simulink model "TEST_IPM_2_0"  (R2019b)
settings: configuration reference "Configuration" (kept outside this file)
PreLoadFcn:
  | RTWConfigurationCB('preloadfcn', bdroot);
values from neighbouring files (symbols this model uses):
  MParamFbase = 200.0    [TEST_IPM_LIB.sldd]
  MParamIbase = 360.0    [TEST_IPM_LIB.sldd]
  MParamLd = 0.002    [TEST_IPM_LIB.sldd]
  MParamLq = 0.002    [TEST_IPM_LIB.sldd]
  MParamRs = 1.15    [TEST_IPM_LIB.sldd]
  PWM_TPBRD_HALF = 5000.0    [TEST_IPM_LIB.sldd]
  Ts_10kHz = 0.0001    [TEST_IPM_LIB.sldd]
  Ts_1kHz = 0.001    [TEST_IPM_LIB.sldd]
undefined symbols (not defined in the file or in its folder): Down, GPTRIP1SEL, GPTRIP2SEL, TZ1, TZ2, Up
libraries: c280xlib x66, c2837xDlib x18, c2802xlib x10, powerlib_meascontrol x9, dsparch4 x4, c2000lib x1, c2806xlib x1, idelinklib_common x1
(part 6 of 6)

== matlab function TEST_IPM_2_0/INT/Extra Observer/MATLAB Function1 ==
  data: idh input; X1_hat output; iqh input; udh input; uqh input; we0 input; weh input; Phid0 input; Phiq0 input; R input; Qx input; QpRs input; QpLdd input; QpLdq input; QpLqq input; X2_hat output; Theta1_hat output; Theta2_hat output; Theta3_hat output; Theta4_hat output; clear input; INITV_RS data_store_memory; INITV_NDQ data_store_memory; INITV_NDD data_store_memory; INITV_NQQ data_store_memory
function [X1_hat,X2_hat,Theta1_hat,Theta2_hat,Theta3_hat,Theta4_hat] = EKF(idh,iqh,udh,uqh,we0,weh,Phid0,Phiq0,R, Qx, QpRs,QpLdd,QpLdq,QpLqq,clear)
global INITV_RS INITV_NDD INITV_NDQ INITV_NQQ
persistent Pk1_k1 Xk1_k1;
if isempty(Pk1_k1)
    Pk1_k1 = single(zeros(6,6));
end
if isempty(Xk1_k1)
    Xk1_k1 = [single(0),single(0),INITV_RS,INITV_NDD,INITV_NDQ,INITV_NQQ]';
end

if(clear ==1)
    Xk1_k1 = [single(0),single(0),INITV_RS,INITV_NDD,INITV_NDQ,INITV_NQQ]';
    Pk1_k1 = single(zeros(6,6));
end
U = [udh;uqh];
Ih= [idh;iqh];
Pk0_k0 = Pk1_k1;
J = single([0,-1;1,0]);
I = single([1,0;0,1]);
Ts = single(1e-4);
Q = single(diag([Qx Qx QpRs QpLdd QpLdq QpLqq]));
R  = [R,0;0,R];
Rs = Xk1_k1(3,1) * I;
T = [Xk1_k1(6,1),Xk1_k1(5,1);...
     Xk1_k1(5,1),Xk1_k1(4,1);];
A = -(we0 * J + Rs * T);
Phi = I + A * Ts + single(0.5) * A^2 * Ts^2;
G = Ts * (I + single(0.5) * A * Ts);
X_hat = [Xk1_k1(1,1);Xk1_k1(2,1)];
X_PE = Phi * X_hat + G * U;
xk1_k0 = [X_PE(1,1);X_PE(2,1);Xk1_k1(3,1);Xk1_k1(4,1);Xk1_k1(5,1);Xk1_k1(6,1);];
Fk0 = [1 + Ts * xk1_k0(3,1) * xk1_k0(6,1),       Ts * (we0 + xk1_k0(3,1) * xk1_k0(5,1)),  Ts * xk1_k0(6,1) * Xk1_k1(1,1) + Ts * xk1_k0(5,1) * Xk1_k1(2,1), 0                             , Ts * xk1_k0(3,1) * Xk1_k1(2,1), Ts * xk1_k0(3,1) * Xk1_k1(1,1);...
       Ts * (-we0 + xk1_k0(3,1) * xk1_k0(5,1)),  1 + Ts * xk1_k0(3,1) * xk1_k0(4,1),      Ts * xk1_k0(5,1) * Xk1_k1(1,1) + Ts * xk1_k0(4,1) * Xk1_k1(2,1), Ts * xk1_k0(3,1) * Xk1_k1(2,1), Ts * xk1_k0(3,1) * Xk1_k1(1,1), 0                             ;...
       0,                                       0,                                      1,                                                               0,                              0,                                0                             ;...
       0,                                       0,                                      0,                                                               1,                              0,                                0                             ;...
       0,                                       0,                                      0,                                                               0,                              1,                                0                             ;...
       0,                                       0,                                      0,                                                               0,                              0,                                1                             ;];
E = Fk0(1:2,1:6) * Pk0_k0;
Temp = [E(1,1)      E(1,2)      E(1,3)      E(1,4)      E(1,5)      E(1,6)      ;...
        E(2,1)      E(2,2)      E(2,3)      E(2,4)      E(2,5)      E(2,6)      ;...
        Pk0_k0(3,1) Pk0_k0(3,2) Pk0_k0(3,3) Pk0_k0(3,4) Pk0_k0(3,5) Pk0_k0(3,6) ;...
        Pk0_k0(4,1) Pk0_k0(4,2) Pk0_k0(4,3) Pk0_k0(4,4) Pk0_k0(4,5) Pk0_k0(4,6) ;...
        Pk0_k0(5,1) Pk0_k0(5,2) Pk0_k0(5,3) Pk0_k0(5,4) Pk0_k0(5,5) Pk0_k0(5,6) ;...
        Pk0_k0(6,1) Pk0_k0(6,2) Pk0_k0(6,3) Pk0_k0(6,4) Pk0_k0(6,5) Pk0_k0(6,6) ;];
Pk1_k0 = Temp * Fk0 + Q;
yk1 = T * X_PE;
yk1Error = Ih - yk1;
Hk = [xk1_k0(6,1),xk1_k0(5,1),0,0,          xk1_k0(2,1),xk1_k0(1,1);...
      xk1_k0(5,1),xk1_k0(4,1),0,xk1_k0(2,1),xk1_k0(1,1),0          ;];
Sk = Hk * Pk1_k0 * Hk' + R;
Kk = Pk1_k0 * Hk' * (Sk^-1);
Xk1_k1 = xk1_k0 + Kk*yk1Error;
Pk1_k1 = (eye(6) - Kk * Hk) * Pk1_k0;

if(Xk1_k1(3,1) > 0.01*100)
    Xk1_k1(3,1) = single(0.01*100);
elseif (Xk1_k1(3,1) < 0.01/100)
    Xk1_k1(3,1) = single(0.01/100);
end
if(Xk1_k1(4,1) > 3.8574*1e3*100)
    Xk1_k1(4,1) = single(3.8574*1e3*100);
elseif (Xk1_k1(4,1) < 3.8574*1e3/100)
    Xk1_k1(4,1) = single(3.8574*1e3/100);
end
if(Xk1_k1(5,1) > 448 * 100)
    Xk1_k1(5,1) =  single(448 * 100);
elseif (Xk1_k1(5,1) <  -448 * 100)
    Xk1_k1(5,1) =  single(-448 * 100);
end
if(Xk1_k1(6,1) > 1.2556*1e4*100)
    Xk1_k1(6,1) = single(1.2556*1e4*100);
elseif (Xk1_k1(6,1) < 1.2556*1e4/100)
    Xk1_k1(6,1) = single(1.2556*1e4/100);
end
X1_hat = Xk1_k1(1,1);X2_hat = Xk1_k1(2,1);
Theta1_hat = Xk1_k1(3,1);Theta2_hat = Xk1_k1(4,1);Theta3_hat = Xk1_k1(5,1);Theta4_hat = Xk1_k1(6,1);

== matlab function TEST_IPM_2_0/INT/Extra Observer/MATLAB Function3 ==
  data: A input; Ldd output; B input; C input; Ldq output; Lqq output
function [Ldd,Ldq,Lqq] = inverse(A,B,C)
T = [C,B;B,A];
V = T^-1;
Ldd = V(1,1);
Ldq = V(1,2);
Lqq = V(2,2);
end

== matlab function TEST_IPM_2_0/CLATask/MATLAB Function5 ==
  data: Ual input; IalEstOut output; Ube input; Ial input; Ibe input; IalEst input; IbeEst input; EalEst input; EbeEst input; LdRated input; LqRated input; RsRated input; we input; K input; eta input; SatPsi input; IbeEstOut output; EalEstOut output; EbeEstOut output
function [IalEstOut,IbeEstOut,EalEstOut,EbeEstOut] = FSO_EEMF(Ual,Ube,Ial,Ibe,IalEst,IbeEst,EalEst,EbeEst,LdRated,LqRated,RsRated,we,K,eta,SatPsi)
sign_al = IalEst - Ial;
sign_be = IbeEst - Ibe;
Ts = single(1e-4);

if(sign_al > single(SatPsi))
    sign_al = single(1);
elseif(sign_al < -single(SatPsi))
    sign_al = -single(1);
else
    sign_al = sign_al * single(1)/single(SatPsi);
end

if(sign_be > single(SatPsi))
    sign_be = single(1);
elseif(sign_be < -single(SatPsi))
    sign_be = -single(1);
else
    sign_be = sign_be * single(1)/single(SatPsi);
end
Temp1 = we * (LdRated - LqRated);
Temp2 = single(1) / LdRated;
% IalEstDot = single(1) / LdRated * (Ual - RsRated * IalEst - we * (LdRated - LqRated) * IbeEst - EalEst + K * sign_al);
% IbeEstDot = single(1) / LdRated * (Ube - RsRated * IbeEst + we * (LdRated - LqRated) * IalEst - EbeEst + K * sign_be);
%%report an error for code too long??
IalEstDot = Ual - RsRated * IalEst - Temp1 * IbeEst;
IalEstDot = IalEstDot - EalEst + K * sign_al;
IalEstDot = IalEstDot * Temp2;

IbeEstDot = Ube - RsRated * IbeEst + Temp1 * IalEst;
IbeEstDot = IbeEstDot - EbeEst + K * sign_be;
IbeEstDot = IbeEstDot * Temp2;

% T = K * [eta,we;-we,eta];
TempEal = eta * sign_al + we * sign_be;
TempEbe = -we  * sign_al + eta * sign_be;
EalEstDot =  - we * EbeEst + K * TempEal;
EbeEstDot =  we * EalEst + K * TempEbe;
% EalEstDot = - we * EbeEst + K * (eta * sign_al + we * sign_be);
% EbeEstDot =   we * EalEst + K * (-we  * sign_al + eta * sign_be);

IalEstOut = IalEst + IalEstDot * Ts;
IbeEstOut = IbeEst + IbeEstDot * Ts;

EalEstOut = EalEst + EalEstDot * Ts;
EbeEstOut = EbeEst + EbeEstDot * Ts;
end

== matlab function TEST_IPM_2_0/INT/Motor Control/Current_PI/RealVoltageCompesation /Subsystem/MATLAB Function3 ==
  data: Eal input; Theta output; Ebe input; ControlAng input; Error output; Eam output
function [Theta,Error,Eam] = atan2(Eal,Ebe, ControlAng)

Theta = atan2(-Eal,Ebe);
if Theta < 0
    Theta = Theta + single(2) * single(pi);
end
Eam = (Eal * Eal + Ebe * Ebe)^(single(0.5));
Error = Theta - ControlAng;
if(Error > single(pi))
    Error = Error - single(2) * single(pi);
elseif(Error < -single(pi))
    Error = Error + single(2) * single(pi);
end

== matlab function TEST_IPM_2_0/SpeedREF/MATLAB Function1 ==
  data: theta input; speed output single; theta_old input; Ts_1kHz parameter
function speed = Est_Speed(theta,theta_old, Ts_1kHz)

error = (theta - theta_old);
if(error > pi)
    error = error - single(2)*single(pi);
elseif(error <- pi)
	error = error + single(2)*single(pi);
end
speed = error/(Ts_1kHz)*single(9.54929674)*single(0.2);
end

== matlab function TEST_IPM_2_0/CLATask/MATLAB Function8 ==
  data: FLAG input
  events: SMOClear output FUNCTION_CALL_EVENT; SMO_V output FUNCTION_CALL_EVENT
function SMO_ENABLE(FLAG)
    if(FLAG == uint16(0))
        SMOClear();
    elseif(FLAG == uint16(2))
        SMO_V();
    end
end

== matlab function TEST_IPM_2_0/INT/Data Buffer/MATLAB Function1 ==
  events: INTFunc output FUNCTION_CALL_EVENT
function START
INTFunc();
end

== matlab function TEST_IPM_2_0/INT/Read Rotor Position/MATLAB Function1 ==
  events: FunCall output FUNCTION_CALL_EVENT
function SpeedDivder
persistent Tick
if isempty(Tick)
    Tick = uint16(0);
end
Tick = Tick + uint16(1);
if(Tick == 10)
    Tick = uint16(0);
    FunCall;
end

== matlab function TEST_IPM_2_0/INT/Read Rotor Position/SpeedCal1/MATLAB Function1 ==
  data: theta input; speed output single; theta_old input; Ts_1kHz parameter
function speed = Est_Speed(theta,theta_old, Ts_1kHz)

error = (theta - theta_old);
if(error > pi)
    error = error - single(2)*single(pi);
elseif(error <- pi)
	error = error + single(2)*single(pi);
end
speed = error/(Ts_1kHz)*single(9.54929674);
end

== matlab function TEST_IPM_2_0/INT/Motor Control/SpeedMode/Function-Call Subsystem/MATLAB Function ==
  data: FLAG input
  events: FcnCal output FUNCTION_CALL_EVENT
function  Action(FLAG)
if(FLAG == uint16(1))
    FcnCal();
end

== matlab function TEST_IPM_2_0/INT/Motor Control/SpeedMode/MATLAB Function1 ==
  data: ThetaEst input; ThetaOut output; FLAG input; ThetaReal input; nREF input
function ThetaOut = ThetaSwitch(ThetaEst,FLAG,ThetaReal,nREF)
if(FLAG == uint16(1))
    ThetaOut = ThetaEst;
elseif(FLAG == uint16(2))
    if(nREF <= single(3.6))
        ThetaOut = ThetaEst;
    else
        ThetaOut = ThetaReal;
    end
else
    ThetaOut = ThetaReal;
end

== matlab function TEST_IPM_2_0/INT/Extra Observer/MATLAB Function7 ==
  data: igamma input; RsOut output; idelta input; ugamma input; udelta input; we0 input; weh input; INITV_RS data_store_memory; INITV_NDD data_store_memory; INITV_NDQ data_store_memory; INITV_NQQ data_store_memory; INITV_PSI data_store_memory; DEKF_R input; DEKF_Qx input; DEKF_QpRs input; DEKF_QpNdd input; DEKF_QpNdq input; DEKF_QpNqq input; DEKF_PSI input; DEKF_CLEAR input; LdOut output; LqOut output; PsidmOut output
function [RsOut,LdOut,LqOut,PsidmOut] = DEKF_ParamObSensorless(igamma,idelta,ugamma,udelta,we0,weh,DEKF_R,DEKF_Qx,DEKF_QpRs,DEKF_QpNdd,DEKF_QpNdq,DEKF_QpNqq,DEKF_PSI,DEKF_CLEAR)
global INITV_RS INITV_NDD INITV_NDQ INITV_NQQ INITV_PSI

persistent hat_x hat_param P_hat_x P_hat_param;
persistent difx_difparam K_xk_1 difH_difparam;
if isempty(hat_x)
    hat_x = single([0;0;]);
    hat_param = single([INITV_RS;INITV_NDD;INITV_NDQ;INITV_NQQ;INITV_PSI;]);
    P_hat_x = single(zeros(2));
    P_hat_param = single(zeros(5));
    
    difx_difparam = single(zeros(2,5));
    K_xk_1 = single(zeros(2));
    difH_difparam = single(zeros(2,5));
end
u = [ugamma;udelta;];
i = [igamma;idelta;];
Tsim = single(1e-4);
Qx = single([DEKF_Qx,0;0,DEKF_Qx;]);
Qp = single(diag([DEKF_QpRs DEKF_QpNdd DEKF_QpNdq DEKF_QpNqq DEKF_PSI]));
R = single([DEKF_R,0;0,DEKF_R;]);
J = single([0,-1;1,0]);

%Step1:Param Prior Estimation

param_PE = hat_param;

P_param_PE = P_hat_param + Qp;

%Step2: State Prior Estimation

Rs = param_PE(1);
Ngg = param_PE(2); Ngd = param_PE(3); Ndd = param_PE(4);
Psidm = param_PE(5);
we = we0 + weh;
N = [Ngg Ngd;Ngd Ndd;];
A = (Rs * N + we * J);
tilde_theta = 1/2 * atan(-2 * Ngd / (Ndd - Ngg));
dot_x = u - A * hat_x - we * J * Psidm * [cos(tilde_theta);sin(tilde_theta);];
x_PE = hat_x + dot_x * Tsim;

A_dis = eye(2) - A * Tsim;
P_x_PE = A_dis * P_hat_x * A_dis' + Qx;

%step3: State Kalman Gain
K_xk = P_x_PE * N' * (N * P_x_PE * N' + R)^-1;
P_hat_x = (eye(2) - K_xk * N) * P_x_PE;

%Step4: Param Kalman Gain
difhat_x_difparam = difx_difparam - K_xk_1 * difH_difparam;

TempA = we * Psidm * 1/2 * 1/(1 + (-2 * Ngd / (Ndd - Ngg))^2) * 1 / ((Ndd - Ngg)^2);
TempCOS = TempA * cos(tilde_theta); TempSIN = TempA * sin(tilde_theta);
C1 = TempCOS * Ngd;              C2 = TempSIN * Ngd;
C3 = TempCOS * single(-1) * (Ndd - Ngg); C4 = TempSIN * single(-1) * (Ndd - Ngg);
C5 = TempCOS * single(-1) * Ngd;              C6 = TempSIN * single(-1) * Ngd;

difG_difparam     = -Tsim * [Ngg * hat_x(1) + Ngd * hat_x(2), Rs * hat_x(1) + C1, Rs * hat_x(2) + C3, 0 + C5            , -we * sin(tilde_theta);...
                             Ngd * hat_x(1) + Ndd * hat_x(2), 0             + C2, Rs * hat_x(1) + C4, Rs * hat_x(2) + C6,  we * cos(tilde_theta);];
difG_difparam = difG_difparam + A_dis * difhat_x_difparam;
H_pk = [0, hat_x(1), hat_x(2), 0       , 0;...
        0, 0       , hat_x(1), hat_x(2), 0;];
H_pk = H_pk + N * difG_difparam;

K_pk = P_param_PE * H_pk' * (H_pk * P_param_PE * H_pk' + R)^-1;
P_hat_param = (eye(5) - K_pk * H_pk) * P_param_PE;
%step5: State & Param Prediction
hat_x = x_PE + K_xk * (i - N * x_PE);
hat_param = param_PE + K_pk * (i - N * x_PE);

if(hat_param(1) > single(2.0))
    hat_param(1) = single(2.0);
elseif(hat_param(1) < single(0.2))
    hat_param(1) = single(0.2);
end

if(hat_param(2) > single(3.7e3))
    hat_param(2) = single(3.7e3);
elseif(hat_param(2) < single(3.7e1))
    hat_param(2) = single(3.7e1);
end


if(hat_param(3) > single(3.7e2))
    hat_param(3) = single(3.7e2);
elseif(hat_param(3) < -single(3.7e2))
    hat_param(3) = -single(3.7e2);
end


if(hat_param(4) > single(2.0e3))
    hat_param(4) = single(2.0e3);
elseif(hat_param(4) < single(2.0e1))
    hat_param(4) = single(2.0e1);
end

if(hat_param(5) > single(0.1))
    hat_param(5) = single(0.1);
elseif(hat_param(5) < single(0.24))
    hat_param(5) = single(0.24);
end

%Step6: Update the parameter kalman gain
difx_difparam = difG_difparam;
K_xk_1 = K_xk;
difH_difparam = H_pk;

if(DEKF_CLEAR == uint16(1))
    hat_x = single([0;0;]);
    hat_param = single([INITV_RS;INITV_NDD;INITV_NDQ;INITV_NQQ;INITV_PSI;]);
    P_hat_x = single(zeros(2));
    P_hat_param = single(zeros(5));
    
    difx_difparam = single(zeros(2,5));
    K_xk_1 = single(zeros(2));
    difH_difparam = single(zeros(2,5));
end
P =     [cos(tilde_theta) sin(tilde_theta);-sin(tilde_theta) cos(tilde_theta);];
P_inv = [cos(tilde_theta) -sin(tilde_theta);sin(tilde_theta) cos(tilde_theta);];
NOut = [hat_param(2) hat_param(3);hat_param(3) hat_param(4);];
LOut = P_inv * (NOut^-1) * P;
RsOut = hat_param(1);
LdOut = LOut(1,1); LqOut = LOut(2,2);
PsidmOut = hat_param(5);

== matlab function TEST_IPM_2_0/INT/Extra Observer/MATLAB Function8 ==
  data: nRef input; Gamma output; Bias input
function Gamma = GammaComP(nRef,Bias)

Gamma = single(5.819e-6) * nRef + Bias;

== matlab function TEST_IPM_2_0/SpeedREF/MATLAB Function3 ==
  data: nREF input; K output; T output
function [K,T] = SMOParam(nREF)
if(nREF < single(200))
    K = single(-5);
    T = single(-500);
else
    K = (nREF) * single(-0.018) - single(2.120);
    T = (nREF) * single(-0.120) - single(480.0);
end
